simulink model "S_MTET_SF_MPPT_ALG_V1"  (R2017a)
settings: Solver=FixedStepDiscrete  StartTime=0.0  StopTime=10.0  RelTol=1e-3
undefined symbols (not defined in the file or in its folder): Down, GPTRIP1SEL, GPTRIP2SEL, TZ1, TZ2, Up
libraries: c2802xlib x4, c2806xlib x2
settings Model: ExtModeTrigDuration=8  Creator=dricl  LastModifiedBy=dricl
settings OptimizationCC: DefaultUnderspecifiedDataType=single  PassReuseOutputArgsAs=Individual arguments  MaxStackSize=512
settings DebuggingCC: ParameterTunabilityLossMsg=error
settings HardwareCC: ProdBitPerChar=16  ProdBitPerInt=16  ProdBitPerPointer=32  ProdBitPerSizeT=32  ProdBitPerPtrDiffT=32  ProdLargestAtomicInteger=Integer  ProdLargestAtomicFloat=None  ProdWordSize=16  ProdLongLongMode=on  ProdHWDeviceType=Texas Instruments->C2000
settings SFSimCC: MATLABDynamicMemAlloc=off
settings RTWCC: SystemTargetFile=ert.tlc  HardwareBoard=TI Piccolo F2806x  TLCOptions=-aInlineSetEventsForThisBaseRateFcn=TLC_FALSE -aSuppressMultiTaskScheduler=TLC_FALSE -aRateBasedStepFcn=1  TemplateMakefile=ert_default_tmf  Description=Embedded Coder  Toolchain=Texas Instruments Code Composer Studio v5 (C2000)  CodeExecutionProfiling=on  CodeProfilingSaveOptions=AllData  CodeProfilingInstrumentation=on
settings CodeAppCC: ForceParamTrailComments=on  IgnoreCustomStorageClasses=off  OperatorAnnotations=on  SimulinkDataObjDesc=on  SFDataObjDesc=on  MATLABFcnDesc=on  InsertBlockDesc=on  MATLABSourceComments=on
settings ERTTargetCC: CodeReplacementLibrary=TI C28x  MemSecPackage=tic2000demospkg  MemSecFuncExecute=code_ramfuncs

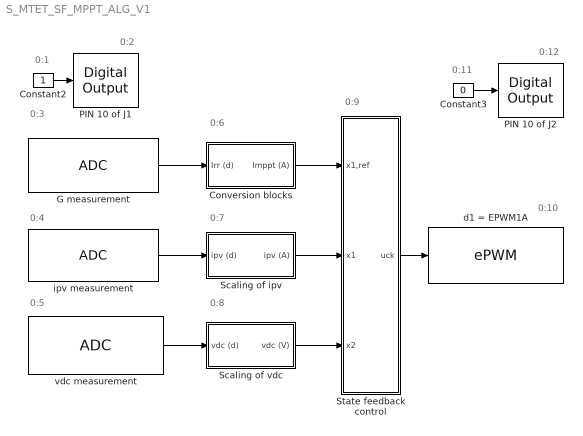
== system S_MTET_SF_MPPT_ALG_V1 ==
  note: 0:1
  note: 0:2
  note: 0:3
  note: 0:4
  note: 0:5
  note: 0:6
  note: 0:7
  note: 0:8
  note: 0:9
  note: 0:10
  note: 0:11
  note: 0:12
  Constant2 : Constant  Priority=1  SampleTime=0.0002
  Constant3 : Constant  Priority=11  Value=0  SampleTime=0.0002
  Conversion blocks : Subsystem  Priority=6  TreatAsAtomicUnit=on
  G measurement : c2802xlib/ADC  Priority=3  ADCModule=1  samplingMode=Single sample mode  ADCResolution=12-bit (Single-ended input)  useSOC1=SOC1  useSOC2=SOC0_SOC1  SOCAcquisitionWindow=7  SOCTriggerSource=ePWM1_ADCSOCA  SOCInterruptTrigger=No ADCINT  Ts=0.0002  dType=uint16  postInterrupt=off  interruptSel=ADCINT1  ADCINTContinuous=on  endma=off  chdma=1  blkParamProc=C2000  conv1=ADCINA1  conv2=ADCINA0 and ADCINB0  conv1_Type4=ADCIN0  conv2_Type4=ADCIN0 and ADCIN1
      settings: SourceProductName=Embedded Coder Support Package for Texas Instruments C2000 Processors
  PIN 10 of J1 : c2806xlib/Digital Output  Priority=2  GPIO_Number=GPIO32~GPIO39  GPIO_Bit0=on  GPIO_BIT0_Toggle=off  GPIO_Bit1=off  GPIO_BIT1_Toggle=off  GPIO_Bit2=off  GPIO_BIT2_Toggle=off  GPIO_Bit3=off  GPIO_BIT3_Toggle=off  GPIO_Bit4=off  GPIO_BIT4_Toggle=off  GPIO_Bit5=off  GPIO_BIT5_Toggle=off  GPIO_Bit6=off  GPIO_BIT6_Toggle=off  GPIO_Bit7=off  GPIO_BIT7_Toggle=off
      settings: SourceProductName=Embedded Coder Support Package for Texas Instruments C2000 Processors  SourceProductBaseCode=TIC2000
  PIN 10 of J2 : c2806xlib/Digital Output  Priority=12  GPIO_Number=GPIO32~GPIO39  GPIO_Bit0=on  GPIO_BIT0_Toggle=off  GPIO_Bit1=off  GPIO_BIT1_Toggle=off  GPIO_Bit2=off  GPIO_BIT2_Toggle=off  GPIO_Bit3=off  GPIO_BIT3_Toggle=off  GPIO_Bit4=off  GPIO_BIT4_Toggle=off  GPIO_Bit5=off  GPIO_BIT5_Toggle=off  GPIO_Bit6=off  GPIO_BIT6_Toggle=off  GPIO_Bit7=off  GPIO_BIT7_Toggle=off
      settings: SourceProductName=Embedded Coder Support Package for Texas Instruments C2000 Processors  SourceProductBaseCode=TIC2000
  Scaling of ipv : Subsystem  Priority=7  TreatAsAtomicUnit=on
  Scaling of vdc : Subsystem  Priority=8  TreatAsAtomicUnit=on
  State feedback control : Subsystem  Priority=9
  d1 = EPWM1A : c2802xlib/ePWM  Priority=10  useModule=ePWM1  ePWMxLINKTBPRD=Not Linked  periodUnits=Clock cycles  timerSource=Specify via dialog  timerPeriod_clk=9000  timerPeriod_sec=0.0001  tbshadow=Counter equals to zero  countingMode=Up-Down  phaseActiveEnable=Disable  phaseDirection=Count down after sync  phaseActive=0  synchronizationEnable=off  dcaevt1Sync=off  dcbevt1Sync=off  synchronizationOption=Disable  clockPrescale=1  HSclockPrescale=1  enswap=off  ePWMxAStatus=on  ePWMxAactionLogic1=Do nothing  ePWMxAactionLogic2=Do nothing  ePWMxAactionLogic3=Clear  ePWMxAactionLogic4=Set  ePWMxAactionLogic5=Do nothing  ePWMxAactionLogic6=Do nothing  ePWMxALoadMode=Load on counter equals to zero (CTR=Zero)  ePWMxACSFenable=off  ePWMxACSFvalue=Forcing disable  ePWMxASFreload=Zero  ePWMxBStatus=off  ePWMxBactionLogic1=Set  ePWMxBactionLogic2=Clear  ePWMxBactionLogic3=Do nothing  ePWMxBactionLogic4=Do nothing  ePWMxBactionLogic5=Clear  ePWMxBactionLogic6=Set  ePWMxBLoadMode=Load on counter equals to zero (CTR=Zero)  ePWMxBCSFenable=off  ePWMxBCSFvalue=Forcing disable  ePWMxBSFreload=Zero  ePWNxBOutWay=off  ePWMxLINKCMPA=Not Linked  CMPAUnits=Clock cycles  CMPASource=Input port  CMPAValue_per=50  CMPAValue_clk=4500  enCMPAshadow=Counter equals to zero  ePWMxLINKCMPB=Not Linked  CMPBUnits=Clock cycles  CMPBSource=Specify via dialog  CMPBValue_per=50  CMPBValue_clk=4500  enCMPBshadow=Counter equals to zero  ePWMxLINKCMPC=Not Linked  CMPCUnits=Clock cycles  CMPCSource=Specify via dialog  CMPCValue_per=50  CMPCValue_clk=32000  enCMPCshadow=Counter equals to zero  ePWMxLINKCMPD=Not Linked  CMPDUnits=Clock cycles  CMPDSource=Specify via dialog  CMPDValue_per=50  CMPDValue_clk=32000  enCMPDshadow=Counter equals to zero  enableDBePWMxA=on  enableDBePWMxB=on  enhalfcycle=off  DBpolarity=Active high complementary (AHC)  DBedgeDelay=Positive  DBSource_ePWMxA=ePWMxA  DBSource_ePWMxB=ePWMxA  DBperiodSource=Specify via dialog  REDperiod=50  FEDperiod=50  adcstartModuleA=on  adcrequestEventA=First event  adcstartEventA=Counter equals to period (CTR=PRD)  adcstartEventA_type2=Digital Compare Module A Event 1 start of conversion (DCAEVT1.soc)  adcstartModuleB=off  adcrequestEventB=First event  adcstartEventB=Counter equals to zero (CTR=Zero)  adcstartEventB_type2=Counter equals to zero (CTR=Zero)  intEn=off  intPrd=First event  intSel=Counter equals to zero (CTR=Zero)  intSel_type2=Counter equals to zero (CTR=Zero)  hrpe=off  enHRPWM=off  HRPWM_LoadMode=Counter equals to period (CTR=PRD)  HRPWM_CTLMode=Duty or Period control mode  HRPWM_EDGMode=Both edge  hrpeb=off  enHRPWMB=off  HRPWM_LoadModeB=Counter equals to zero (CTR=ZERO)  HRPWM_CTLModeB=Duty or Period control mode  HRPWM_EDGModeB=Both edge  enSFO=on  enautoconv=on  chopperEnable=off  chopperFrequency=1  chopperFirstwidth=1  chopperDuty=12.5%  tripZonesource=Specify via dialog  tzselOSHT1=off  tzselOSHT2=off  tzselOSHT3=off  tzselOSHDCAEV1=off  tzselOSHDCBEV1=off  tzselCBC1=off  tzselCBC2=off  tzselCBC3=off  tzselCBCDCAEV2=off  tzselCBCDCBEV2=off  tzselOSHT4=off  tzselOSHT5=off  tzselOSHT6=off  tzselCBC4=off  tzselCBC5=off  tzselCBC6=off  enTzOstIntr=off  enTzCbcIntr=off  enTzDCAEVT1Intr=off  enTzDCAEVT2Intr=off  enTzDCBEVT1Intr=off  enTzDCBEVT2Intr=off  ePWMxAforced=No action  ePWMxBforced=No action  DCAEVT1forced=No action  DCBEVT1forced=No action  DCAEVT2forced=No action  DCBEVT2forced=No action  dcah=Trip Zone 1 input (TZ1)  dcal=Trip Zone 2 input (TZ2)  dcbh=Trip Zone 1 input (TZ1)  dcbl=Trip Zone 2 input (TZ2)  dcah_type2=GPTRIP1SEL/(TZ1)  dcal_type2=GPTRIP2SEL/(TZ2)  dcbh_type2=GPTRIP1SEL/(TZ1)  dcbl_type2=GPTRIP2SEL/(TZ2)  gendcaevt1=Event disabled  gendcaevt2=Event disabled  gendcbevt1=Event disabled  gendcbevt2=Event disabled  dcaevt1src=DCAEVT1 with sync  dcaevt2src=DCAEVT2 with sync  dcbevt1src=DCBEVT1 with sync  dcbevt2src=DCBEVT2 with sync  pulsesel=Counter equals to zero (CTR=Zero)  blankinv=off  blankoffset=0  blankwidth=0  evsrcsel=Filtered version of DCAEVT1 (DCAEVT1FILT)  encape=off  PwmType=C2000
      settings: SourceProductName=Embedded Coder Support Package for Texas Instruments C2000 Processors
  ipv measurement : c2802xlib/ADC  Priority=4  ADCModule=1  samplingMode=Single sample mode  ADCResolution=12-bit (Single-ended input)  useSOC1=SOC2  useSOC2=SOC0_SOC1  SOCAcquisitionWindow=7  SOCTriggerSource=ePWM1_ADCSOCA  SOCInterruptTrigger=No ADCINT  Ts=0.0002  dType=uint16  postInterrupt=off  interruptSel=ADCINT1  ADCINTContinuous=on  endma=off  chdma=1  blkParamProc=C2000  conv1=ADCINA0  conv2=ADCINA0 and ADCINB0  conv1_Type4=ADCIN0  conv2_Type4=ADCIN0 and ADCIN1
      settings: SourceProductName=Embedded Coder Support Package for Texas Instruments C2000 Processors
  vdc measurement : c2802xlib/ADC  Priority=5  ADCModule=1  samplingMode=Single sample mode  ADCResolution=12-bit (Single-ended input)  useSOC1=SOC3  useSOC2=SOC0_SOC1  SOCAcquisitionWindow=7  SOCTriggerSource=ePWM1_ADCSOCA  SOCInterruptTrigger=No ADCINT  Ts=0.0002  dType=uint16  postInterrupt=off  interruptSel=ADCINT1  ADCINTContinuous=on  endma=off  chdma=1  blkParamProc=C2000  conv1=ADCINA2  conv2=ADCINA0 and ADCINB0  conv1_Type4=ADCIN0  conv2_Type4=ADCIN0 and ADCIN1
      settings: SourceProductName=Embedded Coder Support Package for Texas Instruments C2000 Processors
  wires:
  Scaling of ipv/1(ipv (A)) -> State feedback control/2(x1)
  ipv measurement/1 -> Scaling of ipv/1(ipv (d))
  Conversion blocks/1(Imppt (A)) -> State feedback control/1(x1,ref)
  G measurement/1 -> Conversion blocks/1(Irr (d))
  Constant2/1 -> PIN 10 of J1/1
  Constant3/1 -> PIN 10 of J2/1
  vdc measurement/1 -> Scaling of vdc/1(vdc (d))
  Scaling of vdc/1(vdc (V)) -> State feedback control/3(x2)
  State feedback control/1(uck) -> d1 = EPWM1A/1

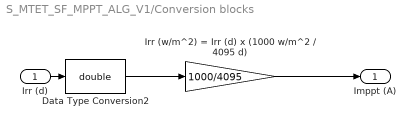
== system S_MTET_SF_MPPT_ALG_V1/Conversion blocks ==
  Irr (d) : Inport
  Data Type Conversion2 : DataTypeConversion  OutDataTypeStr=double
  Irr (w/m^2) = Irr (d) x (1000 w/m^2 / 4095 d) : Gain  Gain=1000/4095
  Imppt (A) : Outport
  wires:
  Irr (d)/1 -> Data Type Conversion2/1
  Data Type Conversion2/1 -> Irr (w/m^2) = Irr (d) x (1000 w/m^2 / 4095 d)/1
  Irr (w/m^2) = Irr (d) x (1000 w/m^2 / 4095 d)/1 -> Imppt (A)/1

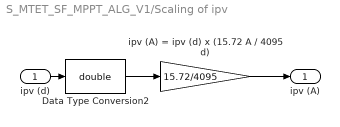
== system S_MTET_SF_MPPT_ALG_V1/Scaling of ipv ==
  ipv (d) : Inport
  Data Type Conversion2 : DataTypeConversion  OutDataTypeStr=double
  ipv (A) = ipv (d) x (15.72 A / 4095 d) : Gain  Gain=15.72/4095
  ipv (A) : Outport
  wires:
  ipv (d)/1 -> Data Type Conversion2/1
  Data Type Conversion2/1 -> ipv (A) = ipv (d) x (15.72 A / 4095 d)/1
  ipv (A) = ipv (d) x (15.72 A / 4095 d)/1 -> ipv (A)/1

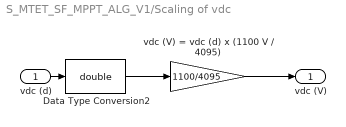
== system S_MTET_SF_MPPT_ALG_V1/Scaling of vdc ==
  vdc (d) : Inport
  Data Type Conversion2 : DataTypeConversion  OutDataTypeStr=double
  vdc (V) = vdc (d) x (1100 V / 4095) : Gain  Gain=1100/4095
  vdc (V) : Outport
  wires:
  Data Type Conversion2/1 -> vdc (V) = vdc (d) x (1100 V / 4095)/1
  vdc (d)/1 -> Data Type Conversion2/1
  vdc (V) = vdc (d) x (1100 V / 4095)/1 -> vdc (V)/1

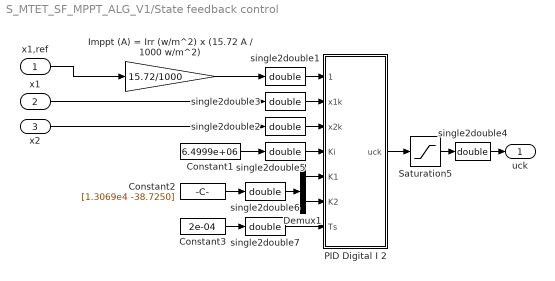
== system S_MTET_SF_MPPT_ALG_V1/State feedback control ==
  x1,ref : Inport
  x1 : Inport  Port=2
  x2 : Inport  Port=3
  Constant1 : Constant  Value=6.4999e+06  SampleTime=2.0000e-04
  Constant2 : Constant  Value=[1.3069e4 -38.7250]  SampleTime=2.0000e-04
  Constant3 : Constant  Priority=10  Value=2e-04  SampleTime=2.0000e-04
  Demux1 : Demux  Outputs=2
  "Imppt (A) = Irr (w/m^2) x (15.72 A / 1000 w/m^2) " : Gain  Gain=15.72/1000
  PID Digital I 2 : MATLAB Function  TreatAsAtomicUnit=on
  Saturation5 : Saturate  UpperLimit=9000*0.98  LowerLimit=9000*0.05
  single2double{1..7} (7 alike) : DataTypeConversion  OutDataTypeStr=double
  uck : Outport
  wires:
  Constant3/1 -> single2double7/1
  PID Digital I 2/1(uck) -> Saturation5/1
  Constant1/1 -> single2double5/1
  Demux1/1 -> PID Digital I 2/5(K1)
  Demux1/2 -> PID Digital I 2/6(K2)
  x1/1 -> single2double3/1
  Saturation5/1 -> single2double4/1
  single2double1/1 -> PID Digital I 2/1(x1k_Ref)
  single2double3/1 -> PID Digital I 2/2(x1k)
  x2/1 -> single2double2/1
  single2double2/1 -> PID Digital I 2/3(x2k)
  single2double4/1 -> uck/1
  single2double5/1 -> PID Digital I 2/4(Ki)
  Constant2/1 -> single2double6/1
  single2double6/1 -> Demux1/1
  single2double7/1 -> PID Digital I 2/7(Ts)
  "Imppt (A) = Irr (w/m^2) x (15.72 A / 1000 w/m^2) "/1 -> single2double1/1
  x1,ref/1 -> "Imppt (A) = Irr (w/m^2) x (15.72 A / 1000 w/m^2) "/1

== matlab function S_MTET_SF_MPPT_ALG_V1/State feedback control/PID Digital I 2 ==
  data: x1k_Ref input; x1k input; x2k input; uck output; Ki input; K1 input; K2 input; Ts input
function uck = fcn(x1k_Ref, x1k, x2k, Ki, K1, K2, Ts)
    % Retroalimentación de estados con acción integral
    
    % Variables persistentes para mantener el estado entre llamadas
    persistent ek Acc_Int Acc_Int_1 uk
    
    if isempty(ek)
        ek = 0;
        Acc_Int = 0;
        Acc_Int_1 = 0;
        uk = 0;
    end

    % Cálculo del error
    ek = x1k_Ref - x1k;

    % Acción integral
    Acc_Int = Ki * ek * Ts + Acc_Int_1;
    Acc_Int_1 = Acc_Int;

    % Ley de control: acción integral menos retroalimentación de estados
    uk = Acc_Int - (K1 * x1k + K2 * x2k);

%     % Saturación (opcional)
%     uk = min(max(uk, 0), 65535);

    % Salida del controlador
    uck = uk;
end
